simulink model "AttitudeINS"  (Simulink 6.6)
settings: Solver=ode4  StartTime=0.0  StopTime=600  FixedStep=SampleT  RelTol=1e-3
InitFcn:
  | clc
  | Taxi_Var
  | failures
  | insInit
values from neighbouring files (symbols this model uses):
  A1 = 0    [Taxi_Var.m]    (also in Taxi_Var_new.m = 0.007)
  Apolar = 0.0899    [Taxi_Var.m]    (also in Taxi_Var_new.m = 0.057)
  APtsamp = 0.005    [failures.m]    (also in piccolo_init.m = 0.05)
  CD0 = 0.0219    [Taxi_Var.m]    (also in Taxi_Var_new.m = 0.022)
  chord = S/span    (= 0.384036716878)    [Taxi_Var.m]    (also in Taxi_Var_new.m = 0.351341681574)
  CL0 = 0.1857    [Taxi_Var.m]    (also in Taxi_Var_new.m = 0.38)
  CLa = 4.6206    [Taxi_Var.m]    (also in Taxi_Var_new.m = 18.5)
  CLa_dot = 1.93    [Taxi_Var.m]    (also in Taxi_Var_new.m = 2.64)
  Clb = -0.0043    [Taxi_Var.m]    (also in Taxi_Var_new.m = -0.06)
  ClDa = 0.1695    [Taxi_Var.m]    (also in Taxi_Var_new.m)
  CLDe = 0.4032    [Taxi_Var.m]    (also in Taxi_Var_new.m = 0.24)
  CLDf = 0.047    [Taxi_Var.m]    (also in Taxi_Var_new.m = 0.4)
  ClDr = 0.0003    [Taxi_Var.m]    (also in Taxi_Var_new.m = 0.055)
  Clp = -0.4425    [Taxi_Var.m]    (also in Taxi_Var_new.m = -0.88)
  CLq = 8.7465    [Taxi_Var.m]    (also in Taxi_Var_new.m = 7.4)
  Clr = 0.0675    [Taxi_Var.m]    (also in Taxi_Var_new.m = 0.04)
  Cm0 = -0.0902    [Taxi_Var.m]    (also in Taxi_Var_new.m = 0.56)
  Cm0_factor = 0.9    [failures.m]
  Cm0_fail = 0    [failures.m]
  Cma = -1.3995    [Taxi_Var.m]    (also in Taxi_Var_new.m = -1.58)
  CmDe = -0.9493    [Taxi_Var.m]    (also in Taxi_Var_new.m = -41)
  CmDf = -.021    (= -0.021)    [Taxi_Var.m]    (also in Taxi_Var_new.m)
  Cnb = 0.0281    [Taxi_Var.m]    (also in Taxi_Var_new.m = 0.73)
  CnDa = -0.0031    [Taxi_Var.m]    (also in Taxi_Var_new.m = -0.032)
  CnDr = -0.0882    [Taxi_Var.m]    (also in Taxi_Var_new.m = 0.19)
  Cnp = -0.0695    [Taxi_Var.m]    (also in Taxi_Var_new.m = -0.1)
  Cnr = -0.1045    [Taxi_Var.m]    (also in Taxi_Var_new.m = -0.23)
  CYb = -0.1999    [Taxi_Var.m]    (also in Taxi_Var_new.m = -0.98)
  CYDr = 0.0192    [Taxi_Var.m]    (also in Taxi_Var_new.m = 0.066)
  da_failamp = 5    [failures.m]
  da_failbias = -da_failamp/2    (= -2.5)    [failures.m]
  da_failper = 90    [failures.m]
  daL_fail = 0    [failures.m]
  daR_fail = 0    [failures.m]
  dr_fail = 0    [failures.m]
  dr_failamp = 2    [failures.m]
  dr_failbias = -dr_failamp/2    (= -1)    [failures.m]
  dr_failper = 70    [failures.m]
  Euler_0 = [0; 0; 45]'*pi/180    [Taxi_Var.m]    (also in Taxi_Var_new.m = [0 0 45]'*pi/180)
  heightDown = 0    [insInit.m]
  heightUp = 3000    [insInit.m]
  ISA_g = 9.815    [Taxi_Var.m]    (also in Taxi_Var_new.m)
  Ixx = 3.689084    [Taxi_Var.m]    (also in Taxi_Var_new.m = 3.8)
  Iyy = 7.43789    [Taxi_Var.m]    (also in Taxi_Var_new.m = 9.58)
  Izz = 10.22202    [Taxi_Var.m]    (also in Taxi_Var_new.m = 9.68)
  latDown = -100000    [insInit.m]
  latUp = 100000    [insInit.m]
  lonDown = -100000    [insInit.m]
  lonUp = 100000    [insInit.m]
  mass = 22.5    [Taxi_Var.m]    (also in Taxi_Var_new.m = 8.16466266)
  MinThK = 0.075    [Taxi_Var.m]    (also in Taxi_Var_new.m = 0.077)
  Pos_0 = [0; 0; 1000]'    [Taxi_Var.m]    (also in Taxi_Var_new.m = [0 0 500]')
  PQR_0 = [0; 0; 0]'    [Taxi_Var.m]    (also in Taxi_Var_new.m = [ 0 0 0]'*pi/180)
  Qk = diag([0.1 0.1 0.1 0.1 0.1 0.1 0.1])    [insInit.m]
  Rk = diag([3 3 5])    [insInit.m]
  SampleT = 0.005    [failures.m]
  span = 2.3368    [Taxi_Var.m]    (also in Taxi_Var_new.m = 2.795)
  tfailure = 20    [failures.m]
  ThK = 2.18    [Taxi_Var.m]    (also in Taxi_Var_new.m = 2.17)
  Vb_0 = [35; 0; 0]'    [Taxi_Var.m]    (also in Taxi_Var_new.m = [35 0 0]')
undefined symbols (not defined in the file or in its folder): clock, DiscIntNeverNeededParam, Earth, gaind, polesd, sigbuilder_block, WGS84, X0, zerosd
libraries: simulink x25, aerolibconvert2 x9, aerolibactuator x6, dspmtrx3 x4, aerolibtransform2 x3, dspsigops x3, aerolibutil x2, aerolibnav x2, dspinverses x1, aerolibatmos2 x1
(part 3 of 3)

== system AttitudeINS/Plant Model/Plant/Forces and Moments/Body Frame F & M/Wind frame F& M/Longitudinal Channel/CL/Lift due to pitch rate ==
  p,q,r : Inport
  Airspeed : Inport  Port=2
  Constant : Constant  Value=CLq
  Get q : Selector  IndexOptions=Index vector (dialog)  Indices=2  OutputSizes=[(-2)]  InputPortWidth=3
  Product : Product  SaturateOnIntegerOverflow=on
  pitch rate factor : Subsystem
  CLq : Outport
  wires:
  pitch rate factor/1(Pitch Rate Fac) -> Product/2
  Constant/1 -> Product/1
  Product/1 -> CLq/1
  p,q,r/1 -> Get q/1
  Get q/1 -> pitch rate factor/1(q)
  Airspeed/1 -> pitch rate factor/2(Airspeed)

== system AttitudeINS/Plant Model/Plant/Forces and Moments/Body Frame F & M/Wind frame F& M/Lateral Channel/Cl/roll factors/roll rate fact ==
  p : Inport
  Airspeed : Inport  Port=2
  Cmq1 : Constant  Value=.5
  Cmq2 : Constant  Value=span
  Product : Product  Inputs=***/  SaturateOnIntegerOverflow=on
  Roll Rate Fac : Outport
  wires:
  Airspeed/1 -> Product/4
  Cmq2/1 -> Product/3
  Cmq1/1 -> Product/2
  p/1 -> Product/1
  Product/1 -> Roll Rate Fac/1

== system AttitudeINS/Plant Model/Plant/Forces and Moments/Body Frame F & M/Wind frame F& M/Lateral Channel/Cl/roll factors/yaw rate fact ==
  r : Inport
  Airspeed : Inport  Port=2
  Cmq1 : Constant  Value=.5
  Cmq2 : Constant  Value=span
  Product : Product  Inputs=***/  SaturateOnIntegerOverflow=on
  Yaw Rate Fac : Outport
  wires:
  Product/1 -> Yaw Rate Fac/1
  Cmq2/1 -> Product/3
  Airspeed/1 -> Product/4
  Cmq1/1 -> Product/2
  r/1 -> Product/1

== system AttitudeINS/Plant Model/Plant/Forces and Moments/Body Frame F & M/Wind frame F& M/Lateral Channel/Cn/yaw factors/roll rate fact ==
  p : Inport
  Airspeed : Inport  Port=2
  Cmq1 : Constant  Value=.5
  Cmq2 : Constant  Value=span
  Product : Product  Inputs=***/  SaturateOnIntegerOverflow=on
  Roll Rate Fac : Outport
  wires:
  Product/1 -> Roll Rate Fac/1
  p/1 -> Product/1
  Cmq1/1 -> Product/2
  Cmq2/1 -> Product/3
  Airspeed/1 -> Product/4

== system AttitudeINS/Plant Model/Plant/Forces and Moments/Body Frame F & M/Wind frame F& M/Lateral Channel/Cn/yaw factors/yaw rate fact ==
  r : Inport
  Airspeed : Inport  Port=2
  Cmq3 : Constant  Value=.5
  Cmq4 : Constant  Value=span
  Product1 : Product  Inputs=***/  SaturateOnIntegerOverflow=on
  Yaw Rate Fac : Outport
  wires:
  Product1/1 -> Yaw Rate Fac/1
  r/1 -> Product1/1
  Cmq3/1 -> Product1/2
  Cmq4/1 -> Product1/3
  Airspeed/1 -> Product1/4

== system AttitudeINS/Plant Model/Plant/Forces and Moments/Body Frame F & M/Wind frame F& M/Longitudinal Channel/CL/Lift due to pitch rate/pitch rate factor ==
  q : Inport
  Airspeed : Inport  Port=2
  Cmq2 : Constant  Value=chord
  Product : Product  Inputs=**/  SaturateOnIntegerOverflow=on
  Pitch Rate Fac : Outport
  wires:
  Product/1 -> Pitch Rate Fac/1
  q/1 -> Product/1
  Airspeed/1 -> Product/3
  Cmq2/1 -> Product/2

== matlab function Prediction/F_k ==
  data: x input inherited; F_k output inherited; omega input inherited
function F_k  = F(x,omega)
% This block supports an embeddable subset of the MATLAB language.
% See the help menu for details. 

F_k = zeros(7,7);

pqr = omega - x(5:7);

F_k (1:4,1:4) = 0.5*[0        -pqr(1)     -pqr(2)     -pqr(3);
                   pqr(1)   0           pqr(3)      -pqr(2);
                   pqr(2)   -pqr(3)      0           pqr(1);
                   pqr(3)   pqr(2)      -pqr(1)     0];
               
F_k (1:4,5:7) = 0.5*[x(2)   x(3)    x(4);
                     -x(1)  x(4)    -x(3);
                     -x(4)   -x(1)   x(2);
                     x(3)   -x(2)   -x(1)];

== matlab function Prediction/f(x,w) ==
  data: x input inherited; x_dot output inherited; omega input inherited
function x_dot  = f(x,omega)
% This block supports an embeddable subset of the MATLAB language.
% See the help menu for details. 

x_dot = zeros(7,1);

pqr = omega - x(5:7);

x_dot (1:4) = 0.5*[0        -pqr(1)     -pqr(2)     -pqr(3);
                   pqr(1)   0           pqr(3)      -pqr(2);
                   pqr(2)   -pqr(3)      0           pqr(1);
                   pqr(3)   pqr(2)      -pqr(1)     0]*x(1:4);

== matlab function Get Measurement/Interpolate Data/Subsystem/Lagrange Interpolation ==
  data: y3 input inherited; polyCoef output inherited; y2 input inherited; y1 input inherited
function polyCoef = lagrInt(y3, y2, y1)
% This block supports an embeddable subset of the MATLAB language.
% See the help menu for details. 

polyCoef = [0 0 0];
%dotCoef = [0 0];
%ddotCoef = 0;
x1 = -2;
x2 = -1;
x3 = 0;

%(1/(x2-x1)/(x2-x3)*y2+1/(x1-x2)/(x1-x3)*y1+1/(x3-x1)/(x3-x2)*y3)*x^2
%((-x2-x3)/(x1-x2)/(x1-x3)*y1+(-x1-x3)/(x2-x1)/(x2-x3)*y2+(-x1-x2)/(x3-x1)/(x3-x2)*y3)*x
% x2*x3/(x1-x2)/(x1-x3)*y1+x1*x2/(x3-x1)/(x3-x2)*y3+x1*x3/(x2-x1)/(x2-x3)*y2

polyCoef(1) = (1/(x2-x1)/(x2-x3)*y2+1/(x1-x2)/(x1-x3)*y1+1/(x3-x1)/(x3-x2)*y3);
polyCoef(2) = ((-x2-x3)/(x1-x2)/(x1-x3)*y1+(-x1-x3)/(x2-x1)/(x2-x3)*y2+(-x1-x2)/(x3-x1)/(x3-x2)*y3);
polyCoef(3) = x2*x3/(x1-x2)/(x1-x3)*y1+x1*x2/(x3-x1)/(x3-x2)*y3+x1*x3/(x2-x1)/(x2-x3)*y2;

%(2/(x1-x2)/(x1-x3)*y1+2/(x2-x1)/(x2-x3)*y2+2/(x3-x1)/(x3-x2)*y3)*x
%(-x2-x3)/(x1-x2)/(x1-x3)*y1+(-x1-x3)/(x2-x1)/(x2-x3)*y2+(-x1-x2)/(x3-x1)/(x3-x2)*y3

%dotCoef(1) = 2*PolyCoef(1);
%dotCoef(2) = PolyCoef(2);

%ddotCoef = dotCoef(1);

== matlab function Correction/H_k ==
  data: x_k_k input inherited; H_k output inherited
function H_k  = H(x_k_k)
% This block supports an embeddable subset of the MATLAB language.
% See the help menu for details. 
H_k = zeros(3,7);
q = x_k_k(1:4);

% Declare the intermediate variables
a = 2*(q(1)*q(2) + q(3)*q(4));
c = 1 - 2*(q(2)^2+ q(3)^2);
gamma = -2*(q(2)*q(4) - q(1)*q(3));
alpha = 2*(q(2)*q(3) + q(1)*q(4));
beta  = 1 - 2*(q(3)^2 + q(4)^2);

% Replace the values
H_k(1,1:4) =          (2*c/(a^2+c^2))*[q(2)     q(1)+2*q(2)*a   q(4)+2*q(3)*a       q(3)];
H_k(2,1:4) =     (2/(sqrt(1-gamma^2)))*[q(3)     -q(4)           q(1)                -q(2)];
H_k(3,1:4) = (2*beta/(alpha^2+beta^2))*[q(4)     q(3)           q(2)+2*q(3)*alpha   q(1)+ 2*q(4)*alpha];

== matlab function Get Measurement/Interpolate Data/Subsystem/Evaluate Poly ==
  data: clock input inherited; polyCoef input inherited; intData output inherited; dotData output inherited; ddotData output inherited
function [intData,dotData,ddotData] = evalPoly(clock, polyCoef)
% This block supports an embeddable subset of the MATLAB language.
% See the help menu for details. 
%clock = clock +1;
intData = polyCoef(1)*clock^2 + polyCoef(2)*clock + polyCoef(3);

dotData = 2*polyCoef(1)*clock + polyCoef(2);

ddotData = polyCoef(1);

== matlab function Get Measurement/Interpolate Data/Subsystem1/Evaluate Poly ==
  data: clock input inherited; polyCoef input inherited; intData output inherited; dotData output inherited; ddotData output inherited
function [intData,dotData,ddotData] = evalPoly(clock, polyCoef)
% This block supports an embeddable subset of the MATLAB language.
% See the help menu for details. 
%clock = clock +1;
intData = polyCoef(1)*clock^2 + polyCoef(2)*clock + polyCoef(3);

dotData = 2*polyCoef(1)*clock + polyCoef(2);

ddotData = polyCoef(1);

== matlab function Get Measurement/Interpolate Data/Subsystem1/Lagrange Interpolation ==
  data: y3 input inherited; polyCoef output inherited; y2 input inherited; y1 input inherited
function polyCoef = lagrInt(y3, y2, y1)
% This block supports an embeddable subset of the MATLAB language.
% See the help menu for details. 

polyCoef = [0 0 0];
%dotCoef = [0 0];
%ddotCoef = 0;
x1 = -2;
x2 = -1;
x3 = 0;

%(1/(x2-x1)/(x2-x3)*y2+1/(x1-x2)/(x1-x3)*y1+1/(x3-x1)/(x3-x2)*y3)*x^2
%((-x2-x3)/(x1-x2)/(x1-x3)*y1+(-x1-x3)/(x2-x1)/(x2-x3)*y2+(-x1-x2)/(x3-x1)/(x3-x2)*y3)*x
% x2*x3/(x1-x2)/(x1-x3)*y1+x1*x2/(x3-x1)/(x3-x2)*y3+x1*x3/(x2-x1)/(x2-x3)*y2

polyCoef(1) = (1/(x2-x1)/(x2-x3)*y2+1/(x1-x2)/(x1-x3)*y1+1/(x3-x1)/(x3-x2)*y3);
polyCoef(2) = ((-x2-x3)/(x1-x2)/(x1-x3)*y1+(-x1-x3)/(x2-x1)/(x2-x3)*y2+(-x1-x2)/(x3-x1)/(x3-x2)*y3);
polyCoef(3) = x2*x3/(x1-x2)/(x1-x3)*y1+x1*x2/(x3-x1)/(x3-x2)*y3+x1*x3/(x2-x1)/(x2-x3)*y2;

%(2/(x1-x2)/(x1-x3)*y1+2/(x2-x1)/(x2-x3)*y2+2/(x3-x1)/(x3-x2)*y3)*x
%(-x2-x3)/(x1-x2)/(x1-x3)*y1+(-x1-x3)/(x2-x1)/(x2-x3)*y2+(-x1-x2)/(x3-x1)/(x3-x2)*y3

%dotCoef(1) = 2*PolyCoef(1);
%dotCoef(2) = PolyCoef(2);

%ddotCoef = dotCoef(1);

== matlab function Get Measurement/Interpolate Data/Subsystem2/Evaluate Poly ==
  data: clock input inherited; polyCoef input inherited; intData output inherited; dotData output inherited; ddotData output inherited
function [intData,dotData,ddotData] = evalPoly(clock, polyCoef)
% This block supports an embeddable subset of the MATLAB language.
% See the help menu for details. 
%clock = clock +1;
intData = polyCoef(1)*clock^2 + polyCoef(2)*clock + polyCoef(3);

dotData = 2*polyCoef(1)*clock + polyCoef(2);

ddotData = polyCoef(1);

== matlab function Get Measurement/Interpolate Data/Subsystem2/Lagrange Interpolation ==
  data: y3 input inherited; polyCoef output inherited; y2 input inherited; y1 input inherited
function polyCoef = lagrInt(y3, y2, y1)
% This block supports an embeddable subset of the MATLAB language.
% See the help menu for details. 

polyCoef = [0 0 0];
%dotCoef = [0 0];
%ddotCoef = 0;
x1 = -2;
x2 = -1;
x3 = 0;

%(1/(x2-x1)/(x2-x3)*y2+1/(x1-x2)/(x1-x3)*y1+1/(x3-x1)/(x3-x2)*y3)*x^2
%((-x2-x3)/(x1-x2)/(x1-x3)*y1+(-x1-x3)/(x2-x1)/(x2-x3)*y2+(-x1-x2)/(x3-x1)/(x3-x2)*y3)*x
% x2*x3/(x1-x2)/(x1-x3)*y1+x1*x2/(x3-x1)/(x3-x2)*y3+x1*x3/(x2-x1)/(x2-x3)*y2

polyCoef(1) = (1/(x2-x1)/(x2-x3)*y2+1/(x1-x2)/(x1-x3)*y1+1/(x3-x1)/(x3-x2)*y3);
polyCoef(2) = ((-x2-x3)/(x1-x2)/(x1-x3)*y1+(-x1-x3)/(x2-x1)/(x2-x3)*y2+(-x1-x2)/(x3-x1)/(x3-x2)*y3);
polyCoef(3) = x2*x3/(x1-x2)/(x1-x3)*y1+x1*x2/(x3-x1)/(x3-x2)*y3+x1*x3/(x2-x1)/(x2-x3)*y2;

%(2/(x1-x2)/(x1-x3)*y1+2/(x2-x1)/(x2-x3)*y2+2/(x3-x1)/(x3-x2)*y3)*x
%(-x2-x3)/(x1-x2)/(x1-x3)*y1+(-x1-x3)/(x2-x1)/(x2-x3)*y2+(-x1-x2)/(x3-x1)/(x3-x2)*y3

%dotCoef(1) = 2*PolyCoef(1);
%dotCoef(2) = PolyCoef(2);

%ddotCoef = dotCoef(1);

== matlab function Get Measurement/Embedded MATLAB Function ==
  data: psi input inherited; Agps input inherited; R output inherited
function R = getR(psi, Agps)
% This block supports an embeddable subset of the MATLAB language.
% See the help menu for details. 

R = [0 0 0];

R(1) = -(cos(psi)*Agps(1) + sin(psi)*Agps(2));
R(2) = -(-sin(psi)*Agps(1) + cos(psi)*Agps(2));
R(3) = 9.81 - Agps(3);

== matlab function Get Measurement/Embedded MATLAB Function1 ==
  data: R input inherited; A input inherited; phi output inherited; theta output inherited
function [phi,theta] = getRP(R, A)
% This block supports an embeddable subset of the MATLAB language.
% See the help menu for details. 

% S = [S_r S_theta S_phi]

S_theta = (R(1)*A(1) + R(3)*sqrt(R(1)^2+R(3)^2-A(1)^2))/(R(1)^2+R(3)^2);
theta = atan2(S_theta*R(1)-A(1), S_theta*R(3));

S_r = R(1)*sin(theta) + R(3)*cos(theta);

S_phi = (R(2)*A(2) + S_r*sqrt(R(2)^2+S_r^2-A(2)^2))/(R(2)^2 + S_r^2);

phi = atan2(-S_phi*R(2) + A(2), S_phi*S_r);
